simulink model "Simulink_EbolaL"  (R2021b)
settings: Solver=VariableStepAuto  StartTime=0.0  StopTime=10.0  FixedStep=0.00126939799450362  RelTol=1e-3
model workspace (MAT data in the model file):
  Beta = 1.89e-07
  C = 8
  Delta = 0.0055
  P = 378
  U = 500
  Uu = 250
  V0 = 1.05
  u = 250
settings Model: Creator=Camilo  LastModifiedBy=Camilo
settings DataIOCC: SaveFormat=Array  OutputTimes=tout

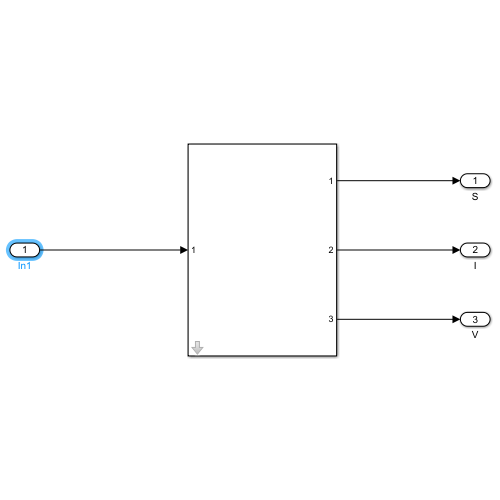
[thumbnail: Simulink's stored preview of the top-level diagram]
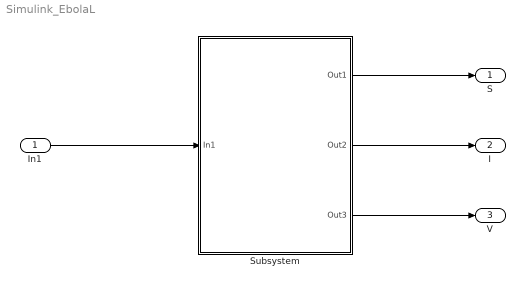
== system Simulink_EbolaL ==
  In1 : Inport
  Subsystem : Subsystem  mask{V0=1, Delta=1e-3, P=378, C=8.02, Beta=1.91e-7}
  S : Outport
  I : Outport  Port=2
  V : Outport  Port=3
  wires:
  Subsystem/1(Out1) -> S/1
  Subsystem/2(Out2) -> I/1
  Subsystem/3(Out3) -> V/1
  In1/1 -> Subsystem/1(In1)

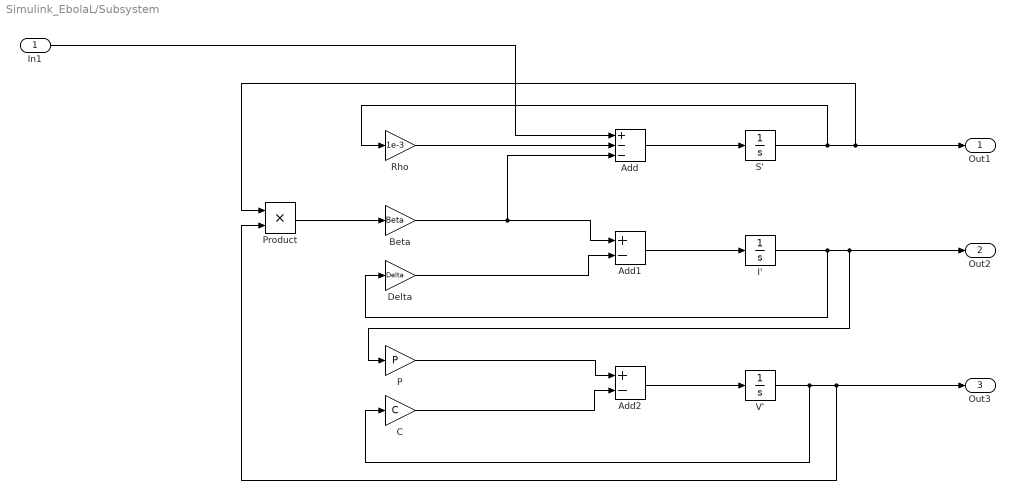
== system Simulink_EbolaL/Subsystem ==
  In1 : Inport
  Add : Sum  Inputs=+--
  Add1 : Sum  Inputs=+-
  Add2 : Sum  Inputs=+-
  Beta : Gain  Gain=Beta
  C : Gain  Gain=C
  Delta : Gain  Gain=Delta
  I' : Integrator  LimitOutput=on  LowerSaturationLimit=0
  P : Gain  Gain=P
  Product : Product
  Rho : Gain  Gain=1e-3
  S' : Integrator  InitialCondition=5e5  LimitOutput=on  LowerSaturationLimit=0
  V' : Integrator  InitialCondition=V0  LimitOutput=on  LowerSaturationLimit=0
  Out1 : Outport
  Out2 : Outport  Port=2
  Out3 : Outport  Port=3
  wires:
  Add/1 -> S'/1
  C/1 -> Add2/2
  Beta/1 -> Add1/1, Add/3
  I'/1 -> Out2/1, P/1, Delta/1
  P/1 -> Add2/1
  S'/1 -> Out1/1, Product/1, Rho/1
  Rho/1 -> Add/2
  V'/1 -> Out3/1, Product/2, C/1
  Add2/1 -> V'/1
  Product/1 -> Beta/1
  Add1/1 -> I'/1
  Delta/1 -> Add1/2
  In1/1 -> Add/1
